simulink model "vacuum_cleaner_simulink"  (R2021a)
settings: Solver=VariableStepAuto  StartTime=0.0  StopTime=10  RelTol=1e-3
undefined symbols (not defined in the file or in its folder): initRoom
libraries: simulink x2
settings Model: Creator=Khaliq Olabintan  LastModifiedBy=Khaliq Olabintan

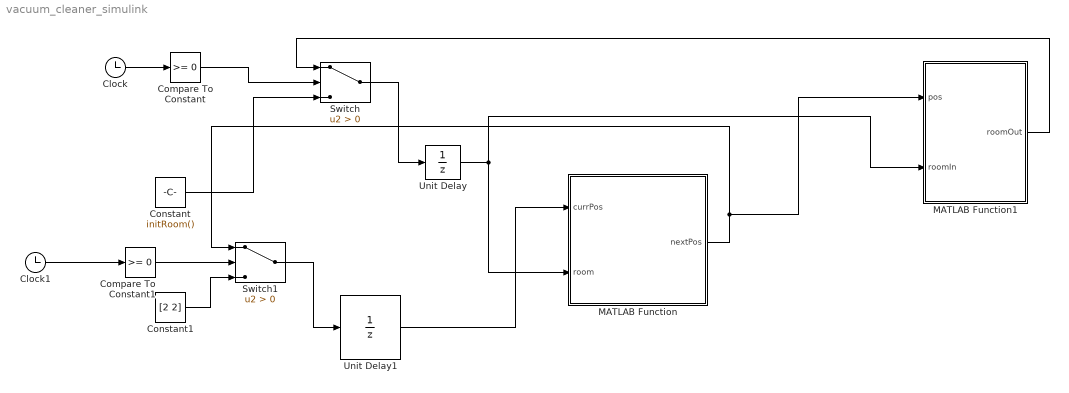
== system vacuum_cleaner_simulink ==
  Clock : Clock
  Clock1 : Clock
  Compare To Constant : simulink/Logic and Bit Operations/Compare To Constant  relop=>=  const=0  OutDataTypeStr=boolean
  Compare To Constant1 : simulink/Logic and Bit Operations/Compare To Constant  relop=>=  const=0  OutDataTypeStr=boolean
  Constant : Constant  Value=initRoom()  OutDataTypeStr=Inherit: Inherit via back propagation
  Constant1 : Constant  Value=[2 2]  OutDataTypeStr=Inherit: Inherit via back propagation
  MATLAB Function : MATLAB Function  TreatAsAtomicUnit=on
  MATLAB Function1 : MATLAB Function  TreatAsAtomicUnit=on
  Switch : Switch  Criteria=u2 > Threshold
  Switch1 : Switch  Criteria=u2 > Threshold
  Unit Delay : UnitDelay  SampleTime=-1  StateName=ROOM MEMORY  HasFrameUpgradeWarning=on
  Unit Delay1 : UnitDelay  SampleTime=-1  HasFrameUpgradeWarning=on
  wires:
  Unit Delay1/1 -> MATLAB Function/1(currPos)
  Unit Delay/1 -> MATLAB Function/2(room), MATLAB Function1/2(roomIn)
  MATLAB Function/1(nextPos) -> Switch1/1, MATLAB Function1/1(pos)
  MATLAB Function1/1(roomOut) -> Switch/1
  Constant/1 -> Switch/3
  Switch/1 -> Unit Delay/1
  Constant1/1 -> Switch1/3
  Switch1/1 -> Unit Delay1/1
  Compare To Constant/1 -> Switch/2
  Compare To Constant1/1 -> Switch1/2
  Clock/1 -> Compare To Constant/1
  Clock1/1 -> Compare To Constant1/1

== matlab function vacuum_cleaner_simulink/MATLAB Function ==
  data: currPos input double size=[1 2]; nextPos output double size=[1 2]; room input double size=[20 20]
function nextPos = robotController(currPos, room)
%#codegen

% Ensure input position is within bounds
rows = size(room, 1);
cols = size(room, 2);
x = max(1, min(rows, currPos(1)));
y = max(1, min(cols, currPos(2)));
currPos = [x, y];

% Get path
path = bfsToNearestDirty(currPos, room);

% Move to next position
if size(path, 1) >= 2
    nextPos = path(2, :);  % Move to next step
else
    nextPos = currPos;     % Stay in place
end
end

% Subfunction: Breadth-First Search
function path = bfsToNearestDirty(startPos, room)
MAX_QUEUE = 1000;
queue = zeros(MAX_QUEUE, 2);
head = 1;
tail = 1;

[rows, cols] = size(room);
visited = zeros(rows, cols);
parent = zeros(rows, cols, 2);

% Direction vectors: right, down, left, up
directions = [0 1; 1 0; 0 -1; -1 0];

% Initialize queue
queue(tail, :) = startPos;
visited(startPos(1), startPos(2)) = 1;
tail = tail + 1;

found = false;
while head < tail
    curr = queue(head, :);
    head = head + 1;

    if room(curr(1), curr(2)) == 1
        % Dirty tile found → backtrack to build path
        path = curr;
        while any(parent(curr(1), curr(2), :))
            prev = [parent(curr(1), curr(2), 1), parent(curr(1), curr(2), 2)];
            path = [prev; path];
            curr = prev;
        end
        found = true;
        return;
    end

    % Expand neighbors
    for i = 1:4
        next = curr + directions(i, :);
        if isValid(next, room, visited)
            queue(tail, :) = next;
            tail = tail + 1;
            visited(next(1), next(2)) = 1;
            parent(next(1), next(2), :) = curr;
        end
    end
end

% Fallback if no path found → just return current position
path = startPos;
end

% Subfunction: Check valid move
function ok = isValid(pos, room, visited)
[rows, cols] = size(room);
x = pos(1);
y = pos(2);
ok = x >= 1 && x <= rows && y >= 1 && y <= cols && ...
     room(x, y) ~= -1 && visited(x, y) == 0;
end

== matlab function vacuum_cleaner_simulink/MATLAB Function1 ==
  data: pos input; roomOut output; roomIn input
function roomOut = mapUpdater(pos, roomIn)
    roomOut = roomIn;
    x = pos(1); y = pos(2);
    if roomOut(x, y) == 1
        roomOut(x, y) = 0;
    end
end
